simulink model "kette1"  (Simulink 4.00)
settings: Solver=ode45  StartTime=0.0  StopTime=10.0  RelTol=1e-3
values from neighbouring files (symbols this model uses):
  g = 9.81    [behaelter_1.m]    (also in behaelter_2.m; kette_1.m = 9.8; pendel_1.m = 9.8; pendel_2.m = 9.8)
  mue = 0.5    [kette_1.m]
  P = 200    [kette_1.m]
  ro = 1000    [behaelter_1.m]    (also in behaelter_2.m; kette_1.m = 10)
  x0 = 0.5    [behaelter_1.m]    (also in behaelter_2.m; kette_1.m = 1; mehrw_3.m = [0 0 0 0 0 1 0 0 0 0]; mehrw_4.m = [0 0 0 0 0 1 0 0 0 0])
settings Model: LastModifiedBy=Administrator  BlockReductionOpt=off

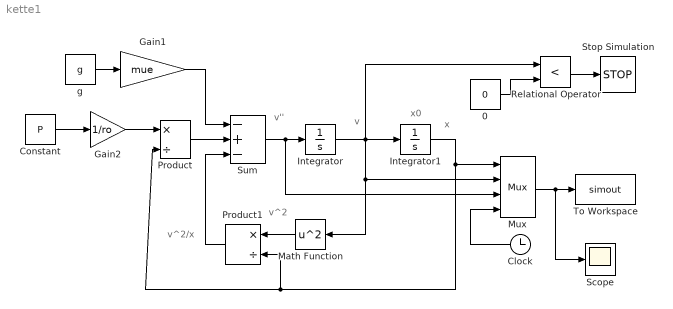
== system kette1 ==
  note: v''
  note: v
  note: x
  note: v^2
  note: v^2/x
  note: x0
  0 : Constant  Value=0
  Clock : Clock
      settings: DisplayTime=off  Decimation=10
  Constant : Constant  Value=P
  Gain1 : Gain  Gain=mue  Multiplication=Element-wise(K.*u)  SaturateOnIntegerOverflow=on
  Gain2 : Gain  Gain=1/ro  Multiplication=Element-wise(K.*u)  SaturateOnIntegerOverflow=on
  Integrator : Integrator  ExternalReset=none  InitialConditionSource=internal  InitialCondition=0  LimitOutput=off  UpperSaturationLimit=inf  LowerSaturationLimit=-inf  ShowSaturationPort=off  ShowStatePort=off  AbsoluteTolerance=auto
  Integrator1 : Integrator  ExternalReset=none  InitialConditionSource=internal  InitialCondition=x0  LimitOutput=off  UpperSaturationLimit=inf  LowerSaturationLimit=-inf  ShowSaturationPort=off  ShowStatePort=off  AbsoluteTolerance=auto
  Math Function : Math  Orientation=left  Operator=square  OutputSignalType=auto
  Mux : Mux  Inputs=4
      settings: DisplayOption=none
  Product : Product  Inputs=*/  Multiplication=Element-wise(.*)  SaturateOnIntegerOverflow=on
  Product1 : Product  Orientation=left  Inputs=*/  Multiplication=Element-wise(.*)  SaturateOnIntegerOverflow=on
  Relational Operator : RelationalOperator  Operator=<
  Scope : Scope
      settings: TimeRange=auto  YMin=-5  YMax=5  SaveToWorkspace=off  SaveName=ScopeData  LimitDataPoints=on  MaxDataPoints=5000
  Stop Simulation : Stop
  Sum : Sum  Inputs=-+-  SaturateOnIntegerOverflow=on
  To Workspace : ToWorkspace  VariableName=simout  SampleTime=-1  SaveFormat=Array
  g : Constant  Value=g
  wires:
  Sum/1 -> Integrator/1, Mux/3
  Integrator/1 -> Integrator1/1, Math Function/1, Mux/2, Relational Operator/1
  Integrator1/1 -> Mux/1, Product/2, Product1/2
  Mux/1 -> To Workspace/1, Scope/1
  Constant/1 -> Gain2/1
  g/1 -> Gain1/1
  Gain2/1 -> Product/1
  Product/1 -> Sum/2
  Math Function/1 -> Product1/1
  Product1/1 -> Sum/3
  Gain1/1 -> Sum/1
  Clock/1 -> Mux/4
  0/1 -> Relational Operator/2
  Relational Operator/1 -> Stop Simulation/1
